simulink model "DFIG_FCS_MPC_sim"  (R2023b)
settings: Solver=ode45  StartTime=0.0  StopTime=1  MaxStep=5e-6  RelTol=1e-3
settings Model: Creator=Y  LastModifiedBy=Y

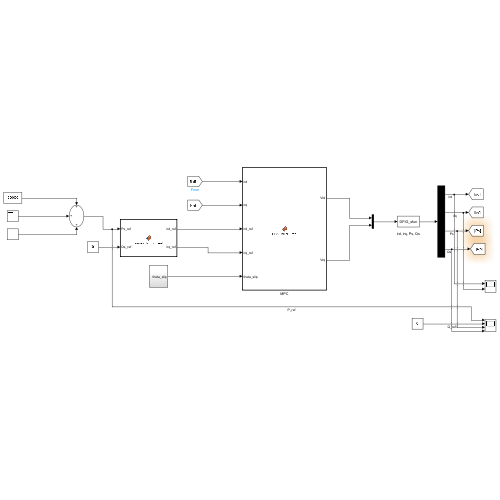
[thumbnail: Simulink's stored preview of the top-level diagram]
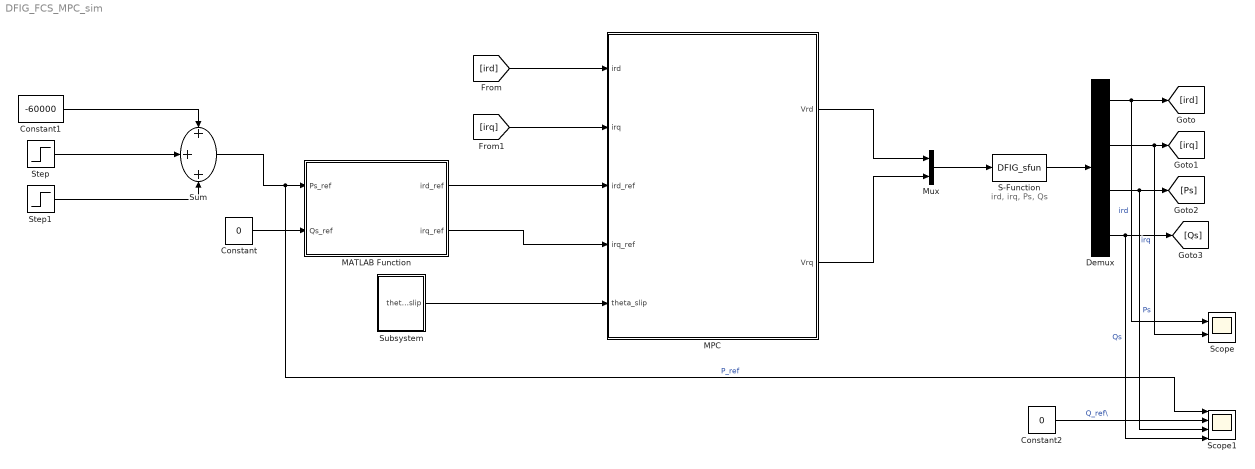
== system DFIG_FCS_MPC_sim ==
  note: ird, irq, Ps, Qs
  Constant : Constant  Value=0
  Constant1 : Constant  Value=-60000
  Constant2 : Constant  Value=0
  Demux : Demux
  MATLAB Function : MATLAB Function  TreatAsAtomicUnit=on
  MPC : MATLAB Function  TreatAsAtomicUnit=on
  Mux : Mux  Inputs=2
  S-Function : S-Function  FunctionName=DFIG_sfun  SFunctionDeploymentMode=off  EnableBusSupport=off
  Scope : Scope  NumInputPorts=2
  Scope1 : Scope  NumInputPorts=4
  Step : Step  Time=0.3  After=-40000  SampleTime=0
  Step1 : Step  Time=0.6  After=-49200  SampleTime=0
  Subsystem : Subsystem
  Sum : Sum  Inputs=+++
  wires:
  Subsystem/1(theta_slip) -> MPC/5(theta_slip)
  MATLAB Function/1(ird_ref) -> MPC/3(ird_ref)
  MATLAB Function/2(irq_ref) -> MPC/4(irq_ref)
  MPC/1(Vrd) -> Mux/1
  MPC/2(Vrq) -> Mux/2
  Mux/1 -> S-Function/1
  S-Function/1 -> Demux/1
  Demux/1 -> Scope/1, [ird]  "ird"
  Demux/4 -> Scope1/4, [Qs]  "Qs"
  Demux/3 -> Scope1/3, [Ps]  "Ps"
  Demux/2 -> Scope/2, [irq]  "irq"
  [irq] -> MPC/2(irq)
  [ird] -> MPC/1(ird)
  Constant/1 -> MATLAB Function/2(Qs_ref)
  Step/1 -> Sum/2
  Step1/1 -> Sum/3
  Constant1/1 -> Sum/1
  Sum/1 -> Scope1/1, MATLAB Function/1(Ps_ref)  "P_ref"
  Constant2/1 -> Scope1/2  "Q_ref\\"

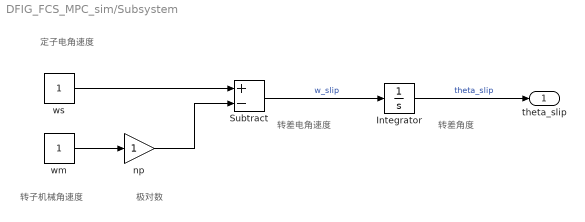
== system DFIG_FCS_MPC_sim/Subsystem ==
  note: 转差角度
  note: 转差电角速度
  note: 极对数
  note: 定子电角速度
  note: 转子机械角速度
  Integrator : Integrator
  Subtract : Sum  Inputs=+-
  np : Gain
  wm : Constant
  ws : Constant
  theta_slip : Outport
  wires:
  ws/1 -> Subtract/1
  Integrator/1 -> theta_slip/1  "theta_slip"
  Subtract/1 -> Integrator/1  "w_slip"
  wm/1 -> np/1
  np/1 -> Subtract/2

== matlab function DFIG_FCS_MPC_sim/MATLAB Function ==
  data: Ps_ref input; ird_ref output; Qs_ref input; irq_ref output
function [ird_ref, irq_ref] = power_to_current(Ps_ref, Qs_ref)
% 功率参考 → 转子电流参考

Ls = 0.03459; Lm = 0.03348;
Vs = 460/sqrt(3); ws = 2*pi*60;
psi_s = Vs / ws;

irq_ref = -Ps_ref * Ls / (1.5 * Lm * Vs);
ird_ref = psi_s / Lm - Qs_ref * Ls / (1.5 * Lm * Vs);
end

== matlab function DFIG_FCS_MPC_sim/MPC ==
  data: ird input; Vrd output; irq input; ird_ref input; irq_ref input; theta_slip input; Vrq output
function [Vrd, Vrq] = FCS_MPC_fcn(ird, irq, ird_ref, irq_ref, theta_slip)
% FCS-MPC 控制器：穷举 8 个矢量，选代价最小的

% 参数
Rr = 0.018; Ls = 0.03459; Lr = 0.03459; Lm = 0.03348;
Np = 2; ws = 2*pi*60; Vs = 460/sqrt(3);
sigma = 1 - Lm^2/(Ls*Lr);
sLr = sigma * Lr;
psi_s = Vs / ws;
wm = 226.6;
w_slip = ws - Np * wm;
Vdc = 800;
Ts = 100e-6;        %采样率是 100 μs

% 8 个开关状态
Sa = [0 1 1 0 0 0 1 1];
Sb = [0 0 1 1 1 0 0 1];
Sc = [0 0 0 0 1 1 1 1];

% Park 变换
ct = cos(theta_slip); st = sin(theta_slip);
ct2 = cos(theta_slip - 2*pi/3); st2 = sin(theta_slip - 2*pi/3);
ct3 = cos(theta_slip + 2*pi/3); st3 = sin(theta_slip + 2*pi/3);

J_min = 1e20;
Vrd_opt = 0;
Vrq_opt = 0;

for j = 1:8
    % abc 相电压
    Sj = [Sa(j); Sb(j); Sc(j)];
    Va = Vdc/3 * (2*Sj(1) - Sj(2) - Sj(3));
    Vb = Vdc/3 * (-Sj(1) + 2*Sj(2) - Sj(3));
    Vc = Vdc/3 * (-Sj(1) - Sj(2) + 2*Sj(3));

    % Park 变换 abc → dq 等幅值变换
    Vrd_j = 2/3 * (Va*ct + Vb*ct2 + Vc*ct3);
    Vrq_j = 2/3 * (-Va*st - Vb*st2 - Vc*st3);

    % 预测
    ird_p = ird + (Ts/sLr) * (Vrd_j - Rr*ird + w_slip*sLr*irq);
    irq_p = irq + (Ts/sLr) * (Vrq_j - Rr*irq - w_slip*(sLr*ird + Lm/Ls*psi_s));

    % 代价函数
    J = (ird_ref - ird_p)^2 + (irq_ref - irq_p)^2;

    if J < J_min
        J_min = J;
        Vrd_opt = Vrd_j;
        Vrq_opt = Vrq_j;
    end
end

Vrd = Vrd_opt;
Vrq = Vrq_opt;
end
